simulink model "test_ekf"  (R2022b)
settings: Solver=FixedStepAuto  StartTime=0.0  StopTime=20.0  FixedStep=0.002  RelTol=1e-3
settings Model: Creator=lucam  LastModifiedBy=ortol

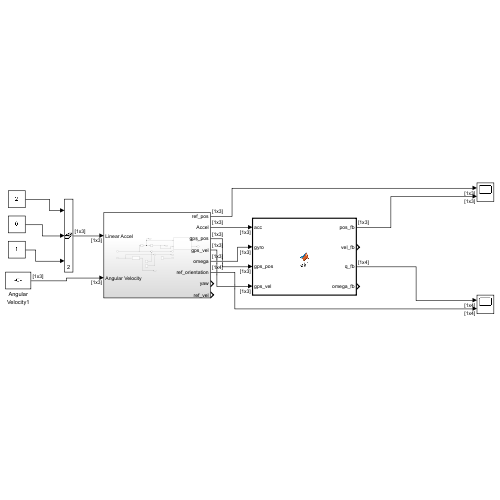
[thumbnail: Simulink's stored preview of the top-level diagram]
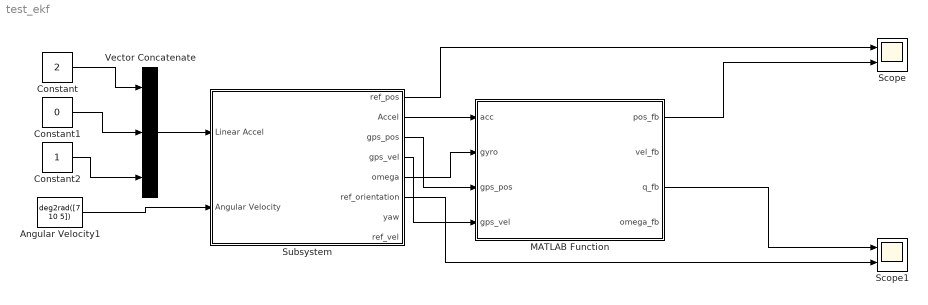
== system test_ekf ==
  Angular Velocity1 : Constant  Value=deg2rad([7 10 5])  VectorParams1D=off  SampleTime=-1
  Constant : Constant  Value=2  SampleTime=0.01
  Constant1 : Constant  Value=0  SampleTime=0.01
  Constant2 : Constant
  MATLAB Function : MATLAB Function  TreatAsAtomicUnit=on
  Scope : Scope  NumInputPorts=2
  Scope1 : Scope  NumInputPorts=2
  Subsystem : Subsystem
  Vector Concatenate : Concatenate  NumInputs=3  Mode=Multidimensional array  ConcatenateDimension=2
  wires:
  Vector Concatenate/1 -> Subsystem/1(Linear Accel)
  Constant1/1 -> Vector Concatenate/2
  Constant/1 -> Vector Concatenate/1
  Constant2/1 -> Vector Concatenate/3
  Angular Velocity1/1 -> Subsystem/2(Angular Velocity)
  Subsystem/2(Accel) -> MATLAB Function/1(acc)
  Subsystem/5(omega) -> MATLAB Function/2(gyro)
  Subsystem/3(gps_pos) -> MATLAB Function/3(gps_pos)
  Subsystem/4(gps_vel) -> MATLAB Function/4(gps_vel)
  Subsystem/1(ref_pos) -> Scope/1
  MATLAB Function/1(pos_fb) -> Scope/2
  MATLAB Function/3(q_fb) -> Scope1/1
  Subsystem/6(ref_orientation) -> Scope1/2

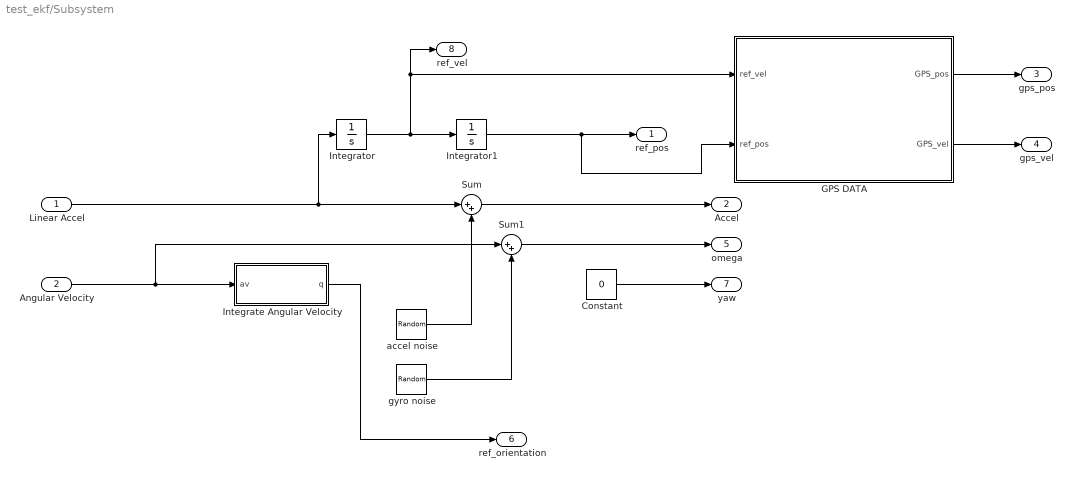
== system test_ekf/Subsystem ==
  Linear Accel : Inport
  Angular Velocity : Inport  Port=2
  Constant : Constant  Value=0
  GPS DATA : Subsystem
  Integrate Angular Velocity : MATLAB Function  TreatAsAtomicUnit=on  mask{rate=100}
      mask prompts: rate "Sample Rate"
  Integrator : Integrator
  Integrator1 : Integrator
  Sum : Sum  Inputs=|++
  Sum1 : Sum  Inputs=|++
  accel noise : RandomNumber  Variance=0
  gyro noise : RandomNumber  Variance=0
  ref_pos : Outport
  Accel : Outport  Port=2
  gps_pos : Outport  Port=3
  gps_vel : Outport  Port=4
  omega : Outport  Port=5
  ref_orientation : Outport  Port=6
  yaw : Outport  Port=7
  ref_vel : Outport  Port=8
  wires:
  Sum1/1 -> omega/1
  Linear Accel/1 -> Sum/1, Integrator/1
  Integrate Angular Velocity/1(q) -> ref_orientation/1
  Integrator/1 -> GPS DATA/1(ref_vel), ref_vel/1, Integrator1/1
  Angular Velocity/1 -> Sum1/1, Integrate Angular Velocity/1(av)
  Integrator1/1 -> GPS DATA/2(ref_pos), ref_pos/1
  GPS DATA/2(GPS_vel) -> gps_vel/1
  GPS DATA/1(GPS_pos) -> gps_pos/1
  Sum/1 -> Accel/1
  accel noise/1 -> Sum/2
  gyro noise/1 -> Sum1/2
  Constant/1 -> yaw/1

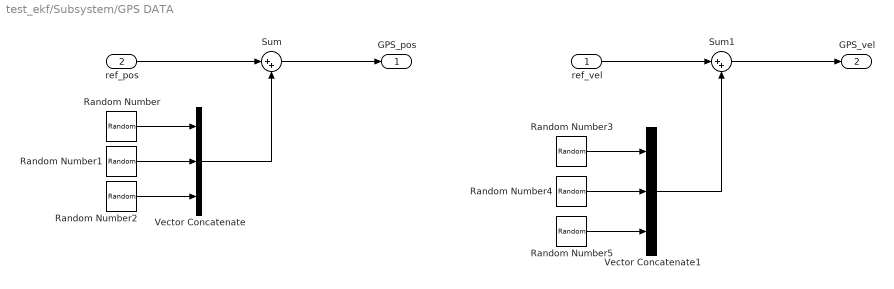
== system test_ekf/Subsystem/GPS DATA ==
  ref_vel : Inport
  ref_pos : Inport  Port=2
  Random Number : RandomNumber  Variance=2
  Random Number1 : RandomNumber  Variance=2
  Random Number2 : RandomNumber  Variance=2
  Random Number3 : RandomNumber  Variance=0.1
  Random Number4 : RandomNumber  Variance=0.1
  Random Number5 : RandomNumber  Variance=0.1
  Sum : Sum  Inputs=|++
  Sum1 : Sum  Inputs=|++
  Vector Concatenate : Concatenate  NumInputs=3  Mode=Multidimensional array  ConcatenateDimension=2
  Vector Concatenate1 : Concatenate  NumInputs=3  Mode=Multidimensional array  ConcatenateDimension=2
  GPS_pos : Outport
  GPS_vel : Outport  Port=2
  wires:
  ref_pos/1 -> Sum/1
  Random Number/1 -> Vector Concatenate/1
  Random Number1/1 -> Vector Concatenate/2
  Random Number2/1 -> Vector Concatenate/3
  Vector Concatenate/1 -> Sum/2
  Sum/1 -> GPS_pos/1
  ref_vel/1 -> Sum1/1
  Random Number3/1 -> Vector Concatenate1/1
  Random Number4/1 -> Vector Concatenate1/2
  Random Number5/1 -> Vector Concatenate1/3
  Vector Concatenate1/1 -> Sum1/2
  Sum1/1 -> GPS_vel/1

== matlab function test_ekf/Subsystem/Integrate Angular Velocity ==
  data: av input; q output; rate parameter
function q = integrateAngVel(av, rate)
%INTEGRATEANGVEL Integrate angular velocity to a quaternion
%  Treat Angular Velocity as an incremental rotation vector.

%   Copyright 2019 The MathWorks, Inc.   

persistent orient
if isempty(orient)
    % Initial orientation is the identity quaternion.
    orient = cast(quaternion(1,0,0,0), 'like', av);
end

% Convert angular velocity to a rotation vector.
rv = quaternion(av*(1/rate), 'rotvec');
orient = rv * orient;
q = compact(orient);

== matlab function test_ekf/MATLAB Function ==
  data: acc input; pos_fb output; gyro input; vel_fb output; q_fb output; omega_fb output; gps_pos input; gps_vel input
function [pos_fb, vel_fb, q_fb, omega_fb] = ekf(acc, gyro, gps_pos, gps_vel)
pos_fb = [0,0,0];
vel_fb = [0,0,0];
q_fb = [1,0,0,0];
omega_fb = [0,0,0];
coder.extrinsic("ekf_mex");
[pos_fb, vel_fb, q_fb, omega_fb] = ekf_mex(acc, gyro, gps_pos, gps_vel);
